simulink model "profinet_simulation_ss_separated"  (R2016b)
settings: Solver=FixedStepAuto  StartTime=0.0  StopTime=80  FixedStep=Ts  RelTol=1e-3
values from neighbouring files (symbols this model uses):
  A = [0 1 0 ... (first row only)    [motor.m]
  B = [0 ; 0 ; 1/L]    [motor.m]
  C = [1 0 0]    [motor.m]
  K = dlqr(Gd.a,Gd.b,diag([1,1,1]),1)    [motor.m]
  Ts = 1e-3    (= 0.001)    [TimeDelayEstimationSearch_Profibus.m]    (also in motor.m = 0.0001)
  Ts_IRT = 1e-4    (= 0.0001)    [motor.m]
  Ts_RT = 1e-3    (= 0.001)    [TimeDelayEstimationSearch_Profibus.m]    (also in motor.m)
  Ts_SRT = 1e-1    (= 0.1)    [motor.m]
libraries: simulink x4
settings Model: Creator=z003vh9b  LastModifiedBy=z003vh9b
settings OptimizationCC: BlockReduction=off  DefaultParameterBehavior=Inlined  BufferReuse=off

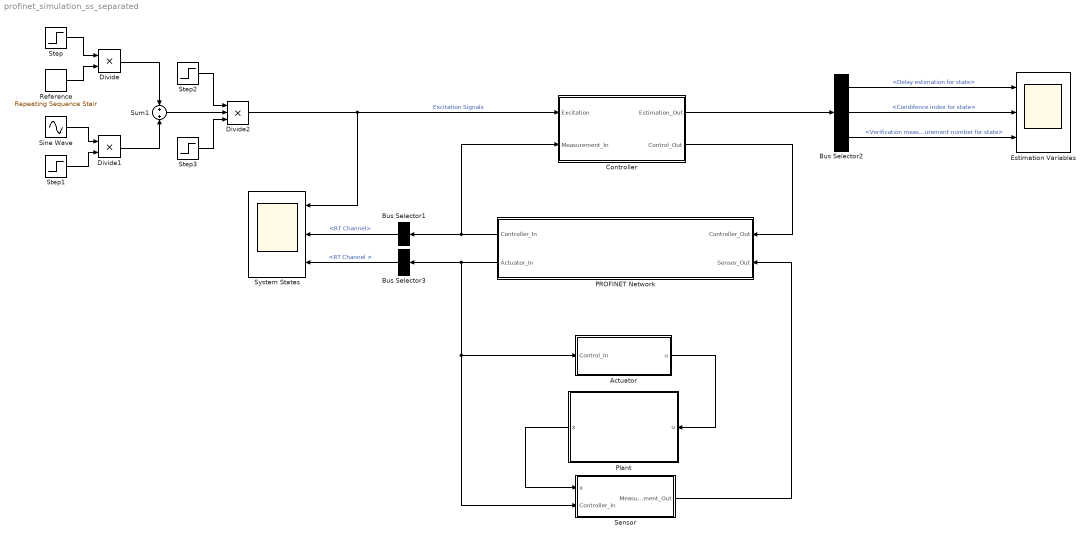
== system profinet_simulation_ss_separated ==
  Actuator : Subsystem  mask(Actuator with PROFIBUS interface){Gain=1, ActuatorCh=RT}
      mask prompts: Gain "Control Gain - Signal Conversion"; ActuatorCh "Control Signal Channel"
      mask help: Actuator Device connected to PROFIBUS network connection.
      mask TypeOptions ActuatorCh: RT | IRT
  Bus Selector1 : BusSelector  OutputSignals=RT Channel
  Bus Selector2 : BusSelector  OutputSignals=Delay estimation for state,Condifence index for state,Verification measurement number for state
  Bus Selector3 : BusSelector  OutputSignals=RT Channel
  Controller : Subsystem  mask(Controller Device with PROFINET Interface){K=K, SensorCh=RT, ActuatorCh=RT, N_ver=90}
      mask prompts: K "Gain"; SensorCh "Sensor measurement Channel"; ActuatorCh "Actuator control Channel"; N_ver "Verification Buffer Size (n samples)"
      mask help: Controller device connected to PROFINET network sending actuator control signals and receiving sensor measurements. Closed loop control is done as State-space optimal control.
      mask TypeOptions SensorCh: RT | IRT
      mask TypeOptions ActuatorCh: RT | IRT
  Divide : Product  Inputs=**
  Divide1 : Product  Inputs=**
  Divide2 : Product  Inputs=***
  Estimation Variables : Scope  NumInputPorts=3
  PROFINET Network : Subsystem  mask(PROFINET network simulation with attacks){PckgLossRate=20, PckgTimeLow=30, PckgTimeUp=90, AttackSensorRT=on, T_RT_Att_Sen=[7.8 2.1 5.04], Val_RT_Att_Sen_init=[0 0 0], Val_RT_Att_Sen=[6 12 10], AttackSensorIRT=off, T_IRT_Att_Sen=0, Val_IRT_Att_Sen_init=0, Val_IRT_Att_Sen=500, AttackControlRT=off, T_RT_Att_Cnt=5, Val_RT_Att_Cnt=3, AttackControlIRT=off, T_IRT_Att_Cnt=3, Val_IRT_Att_Cnt=-2}
      mask prompts: PckgLossRate "Package loss Rate [%]"; PckgTimeLow "Package arival time variation Lower litmit [%] 0-100% Ts"; PckgTimeUp "Package arival time variation Upper litmit [%] 0-100%Ts"; AttackSensorRT "RT Measurement Channel Attack"; T_RT_Att_Sen "Time of the Attack [s]"; Val_RT_Att_Sen_init "Initial Delay Value (n sampling times)"; Val_RT_Att_Sen "Delay Value (n sampling times)"; AttackSensorIRT "IRT Measurement Channel Attack"; T_IRT_Att_Sen "Time of the Attack [s]"; Val_IRT_Att_Sen_init "Initial Delay Value (n sampling times)"; Val_IRT_Att_Sen "Delay Value (n sampling times)"; AttackControlRT "RT Control Channel Attack"; T_RT_Att_Cnt "Time of the Attack [s]"; Val_RT_Att_Cnt "Attack Control Value [V]"; AttackControlIRT "IRT Control Channel Attack"; T_IRT_Att_Cnt "Time of the Attack [s]"; Val_IRT_Att_Cnt "Attack Control Value [V]"
      mask help: This block represents PROFINET network simulaiton with configulable packet loss and time delays. Additionally simulation of Man in the middle cyber attack is provided on both sensor measuremnt side as well as actuator control value.
  Plant : Subsystem  mask(Plant){A=A, B=B, C=C, x0=0}
      mask prompts: A "A Matrix"; B "B Matrix"; C "C Matrix"; x0 "Xo"
      mask help: This dynamical LTI system does not have awareness of PROFINET network. It is formed as continous State-Space domain and all the states can be measured and are provided at the output port (x).
  Reference : simulink/Sources/Repeating Sequence Stair  OutValues=[0 1 2 1 -1].'  tsamp=2  OutMin=[]  OutMax=[]  OutDataTypeStr=double  OutputDataTypeScalingMode=double  OutDataType=fixdt(0,8)  ConRadixGroup=Best Precision: Vector-wise  OutScaling=2^-12
  Sensor : Subsystem  mask(Sensor with PROFIBUS interface){SensorGain=[1 1 1], QuantizationEnable=on, SensorQuantMax=[1 1 1], SensorQuantMin=[-1 -1 -1], SensorQuantN=[2000 2000 2000], SensorNoise=on, NoiseMagnitude=[1e-3 1e-3 1e-3], SensorCh=RT, N_samples=30}
      mask prompts: SensorGain "Sensor Gain - Signal Conversion"; QuantizationEnable "Enable Quantization"; SensorQuantMax "Sensor State Max"; SensorQuantMin "Sensor State Min"; SensorQuantN "Sensor State Quantization - N"; SensorNoise "Enable Smart Noise"; NoiseMagnitude "Smart Noise Unit Magnitude"; SensorCh "Sensor Measurement Channel"; N_samples "Maximal Verification Measurement Number ( n samples )"
      mask help: Sensor Device connected to PROFIBUS network connection. It sends all state variables posible to meassure to the Controller Device.
      mask TypeOptions SensorCh: RT | IRT
      mask DialogControl Control2 Prompt: Sensor states quantiosation (Max-Min)/N
  Sine Wave : Sin  Amplitude=[1 1 1]  Frequency=[70*pi, 60*pi,80*pi]  SampleTime=0
  Step : Step  Time=20  Before=1  After=0  SampleTime=0
  Step1 : Step  Time=40  SampleTime=0
  Step2 : Step  Time=60  Before=1  After=0  SampleTime=0
  Step3 : Step  Time=0  SampleTime=0
  Sum1 : Sum
  System States : Scope  NumInputPorts=3
  wires:
  Actuator/1(u) -> Plant/1(u)
  PROFINET Network/1(Controller_In) -> Controller/2(Measurement_In), Bus Selector1/1
  Plant/1(x) -> Sensor/1(x)
  Controller/2(Control_Out) -> PROFINET Network/1(Controller_Out)
  Sensor/1(Measurement_Out) -> PROFINET Network/2(Sensor_Out)
  PROFINET Network/2(Actuator_In) -> Sensor/2(Controller_In), Actuator/1(Control_In), Bus Selector3/1
  Bus Selector1/1 -> System States/2  "<RT Channel>"
  Controller/1(Estimation_Out) -> Bus Selector2/1
  Bus Selector2/2 -> Estimation Variables/2  "<Condifence index for state>"
  Bus Selector2/1 -> Estimation Variables/1  "<Delay estimation for state>"
  Bus Selector2/3 -> Estimation Variables/3  "<Verification measurement number for state>"
  Bus Selector3/1 -> System States/3  "<RT Channel >"
  Sum1/1 -> Divide2/2
  Sine Wave/1 -> Divide1/1
  Reference/1 -> Divide/2
  Divide1/1 -> Sum1/2
  Divide/1 -> Sum1/1
  Divide2/1 -> Controller/1(Excitation), System States/1  "Excitation Signals"
  Step/1 -> Divide/1
  Step1/1 -> Divide1/2
  Step2/1 -> Divide2/1
  Step3/1 -> Divide2/3

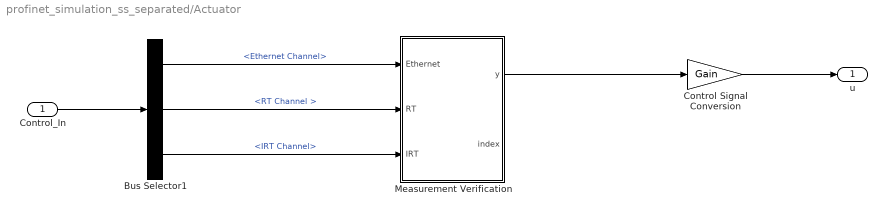
== system profinet_simulation_ss_separated/Actuator ==
  Control_In : Inport
  Bus Selector1 : BusSelector  OutputSignals=Ethernet Channel,RT Channel ,IRT Channel
  Control Signal Conversion : Gain  Gain=Gain
  Measurement Verification : MATLAB Function  TreatAsAtomicUnit=on
  u : Outport
  wires:
  Measurement Verification/1(y) -> Control Signal Conversion/1
  Bus Selector1/3 -> Measurement Verification/3(IRT)  "<IRT Channel>"
  Bus Selector1/1 -> Measurement Verification/1(Ethernet)  "<Ethernet Channel>"
  Control Signal Conversion/1 -> u/1
  Control_In/1 -> Bus Selector1/1
  Bus Selector1/2 -> Measurement Verification/2(RT)  "<RT Channel >"

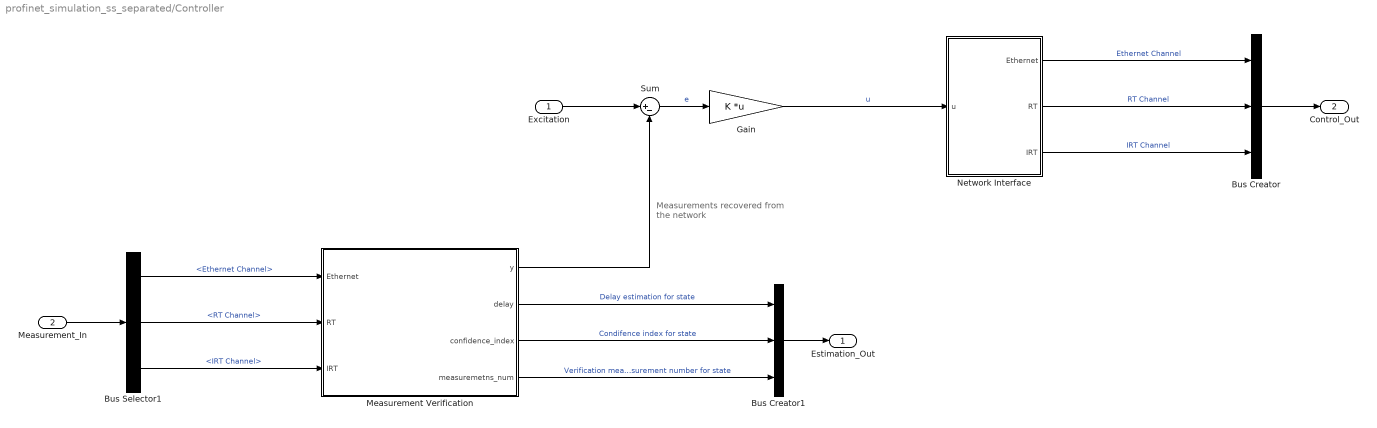
== system profinet_simulation_ss_separated/Controller ==
  note: Measurements recovered
      | from the network
  Excitation : Inport
  Measurement_In : Inport  Port=2
  Bus Creator : BusCreator  Inputs=3
  Bus Creator1 : BusCreator  Inputs=3
  Bus Selector1 : BusSelector  OutputSignals=Ethernet Channel,RT Channel,IRT Channel
  Gain : Gain  Gain=K  Multiplication=Matrix(K*u) (u vector)
  Measurement Verification : MATLAB Function  TreatAsAtomicUnit=on  SystemSampleTime=Ts
  Network Interface : MATLAB Function  TreatAsAtomicUnit=on  SystemSampleTime=Ts
  Sum : Sum  Inputs=|+-
  Estimation_Out : Outport
  Control_Out : Outport  Port=2
  wires:
  Sum/1 -> Gain/1  "e"
  Measurement Verification/1(y) -> Sum/2
  Gain/1 -> Network Interface/1(u)  "u"
  Network Interface/2(RT) -> Bus Creator/2  "RT Channel"
  Bus Selector1/1 -> Measurement Verification/1(Ethernet)  "<Ethernet Channel>"
  Bus Selector1/2 -> Measurement Verification/2(RT)  "<RT Channel>"
  Bus Selector1/3 -> Measurement Verification/3(IRT)  "<IRT Channel>"
  Network Interface/1(Ethernet) -> Bus Creator/1  "Ethernet Channel"
  Network Interface/3(IRT) -> Bus Creator/3  "IRT Channel"
  Measurement Verification/2(delay) -> Bus Creator1/1  "Delay estimation for state"
  Measurement Verification/3(confidence_index) -> Bus Creator1/2  "Condifence index for state"
  Measurement Verification/4(measuremetns_num) -> Bus Creator1/3  "Verification measurement number for state"
  Bus Creator/1 -> Control_Out/1
  Measurement_In/1 -> Bus Selector1/1
  Bus Creator1/1 -> Estimation_Out/1
  Excitation/1 -> Sum/1

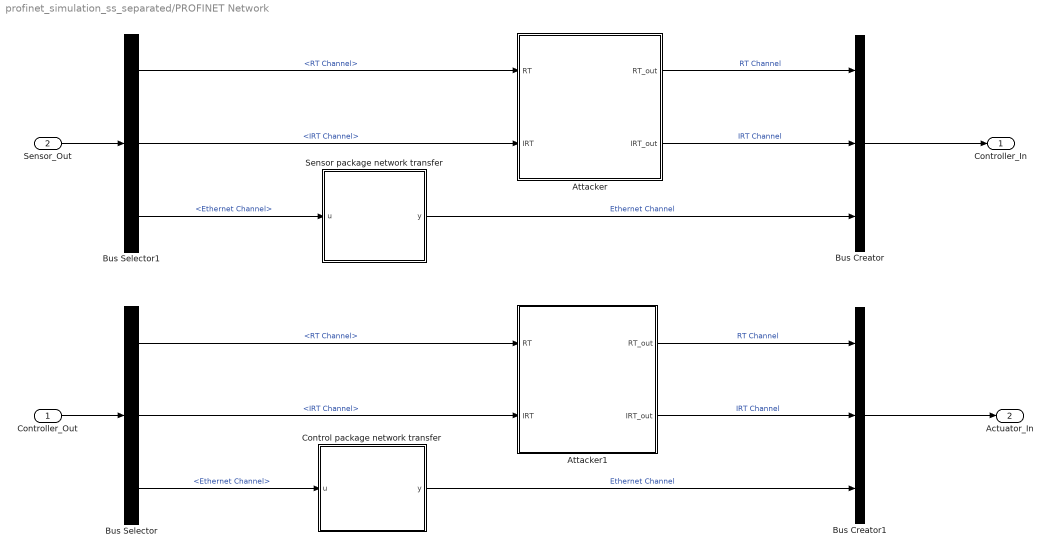
== system profinet_simulation_ss_separated/PROFINET Network ==
  Controller_Out : Inport
  Sensor_Out : Inport  Port=2
  Attacker : Subsystem
  Attacker1 : Subsystem
  Bus Creator : BusCreator  Inputs=3
  Bus Creator1 : BusCreator  Inputs=3
  Bus Selector : BusSelector  OutputSignals=RT Channel,IRT Channel,Ethernet Channel
  Bus Selector1 : BusSelector  OutputSignals=RT Channel,IRT Channel,Ethernet Channel
  Control package network transfer : MATLAB Function  TreatAsAtomicUnit=on
  Sensor package network transfer : MATLAB Function  TreatAsAtomicUnit=on
  Controller_In : Outport
  Actuator_In : Outport  Port=2
  wires:
  Attacker/1(RT_out) -> Bus Creator/1  "RT Channel"
  Attacker1/1(RT_out) -> Bus Creator1/1  "RT Channel"
  Bus Selector/1 -> Attacker1/1(RT)  "<RT Channel>"
  Control package network transfer/1(y) -> Bus Creator1/3  "Ethernet Channel"
  Sensor package network transfer/1(y) -> Bus Creator/3  "Ethernet Channel"
  Controller_Out/1 -> Bus Selector/1
  Bus Selector/3 -> Control package network transfer/1(u)  "<Ethernet Channel>"
  Sensor_Out/1 -> Bus Selector1/1
  Bus Creator/1 -> Controller_In/1
  Bus Creator1/1 -> Actuator_In/1
  Bus Selector1/2 -> Attacker/2(IRT)  "<IRT Channel>"
  Bus Selector1/3 -> Sensor package network transfer/1(u)  "<Ethernet Channel>"
  Bus Selector1/1 -> Attacker/1(RT)  "<RT Channel>"
  Attacker/2(IRT_out) -> Bus Creator/2  "IRT Channel"
  Bus Selector/2 -> Attacker1/2(IRT)  "<IRT Channel>"
  Attacker1/2(IRT_out) -> Bus Creator1/2  "IRT Channel"

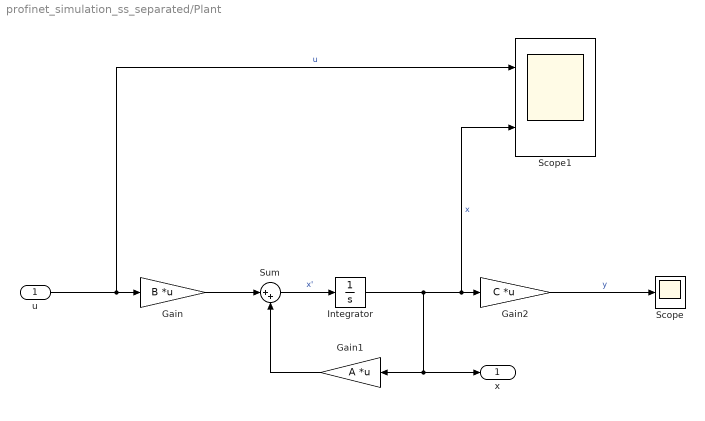
== system profinet_simulation_ss_separated/Plant ==
  u : Inport
  Gain : Gain  Gain=B  Multiplication=Matrix(K*u) (u vector)
  Gain1 : Gain  Gain=A  Multiplication=Matrix(K*u)
  Gain2 : Gain  Gain=C  Multiplication=Matrix(K*u) (u vector)
  Integrator : Integrator  InitialCondition=x0
  Scope : Scope
  Scope1 : Scope  NumInputPorts=2
  Sum : Sum  Inputs=|++
  x : Outport
  wires:
  u/1 -> Scope1/1, Gain/1  "u"
  Integrator/1 -> Gain1/1, x/1, Scope1/2, Gain2/1  "x"
  Gain1/1 -> Sum/2
  Sum/1 -> Integrator/1  "x'"
  Gain/1 -> Sum/1
  Gain2/1 -> Scope/1  "y"

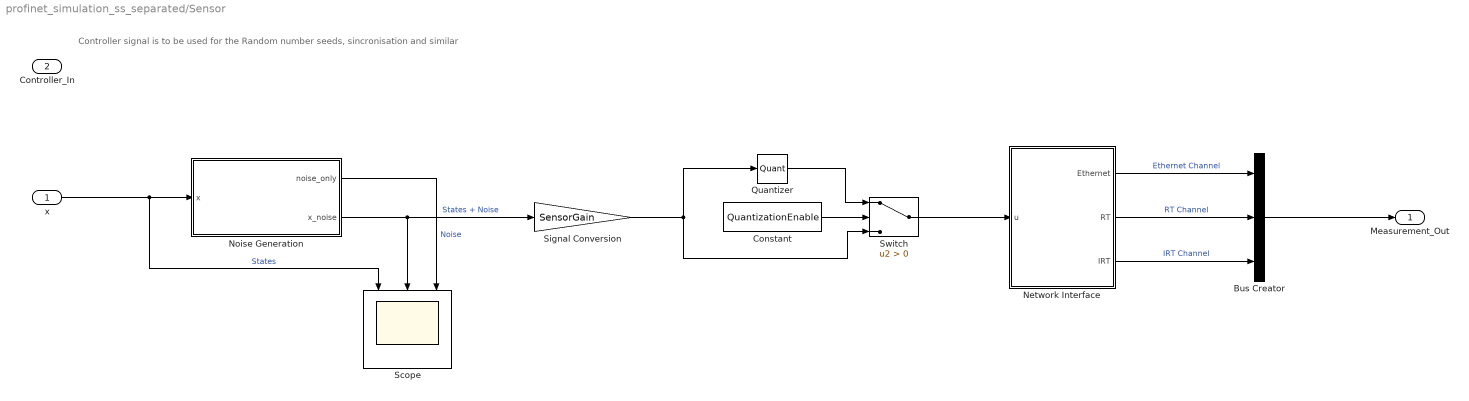
== system profinet_simulation_ss_separated/Sensor ==
  note: Controller signal is to be used for the Random number seeds, sincronisation and similar
  x : Inport
  Controller_In : Inport  Port=2
  Bus Creator : BusCreator  Inputs=3
  Constant : Constant  Value=QuantizationEnable
  Network Interface : MATLAB Function  TreatAsAtomicUnit=on  SystemSampleTime=Ts
  Noise Generation : MATLAB Function  TreatAsAtomicUnit=on  SystemSampleTime=Ts
  Quantizer : Quantizer  QuantizationInterval=(SensorQuantMax-SensorQuantMin)./SensorQuantN
  Scope : Scope  NumInputPorts=3
  Signal Conversion : Gain  Gain=SensorGain
  Switch : Switch  Criteria=u2 > Threshold
  Measurement_Out : Outport
  wires:
  Network Interface/2(RT) -> Bus Creator/2  "RT Channel"
  Network Interface/1(Ethernet) -> Bus Creator/1  "Ethernet Channel"
  Noise Generation/2(x_noise) -> Signal Conversion/1, Scope/2  "States + Noise"
  Network Interface/3(IRT) -> Bus Creator/3  "IRT Channel"
  x/1 -> Noise Generation/1(x), Scope/1  "States"
  Signal Conversion/1 -> Switch/3, Quantizer/1
  Switch/1 -> Network Interface/1(u)
  Quantizer/1 -> Switch/1
  Constant/1 -> Switch/2
  Bus Creator/1 -> Measurement_Out/1
  Noise Generation/1(noise_only) -> Scope/3  "Noise"

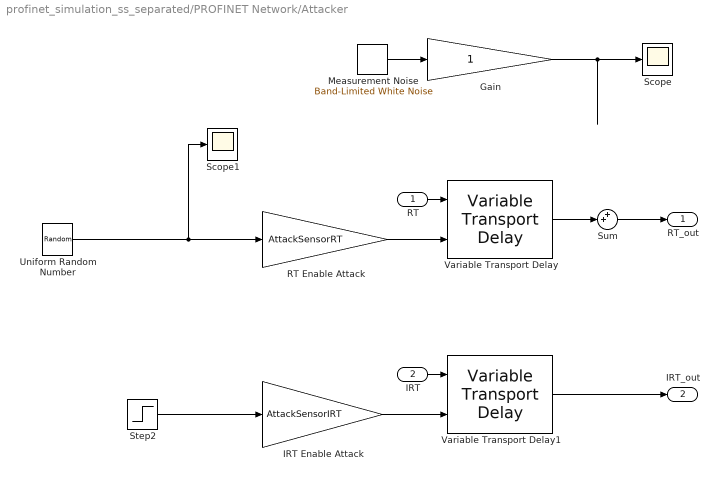
== system profinet_simulation_ss_separated/PROFINET Network/Attacker ==
  RT : Inport  PortDimensions=3
  IRT : Inport  Port=2  PortDimensions=3
  Gain : Gain
  IRT Enable Attack : Gain  Gain=AttackSensorIRT
  Measurement Noise : simulink/Sources/Band-Limited White Noise  Cov=[10e-3,10e-3,10e-3].^2* Ts/(2*pi)  Ts=Ts  seed=[432,23534653441,2353234]
  RT Enable Attack : Gain  Gain=AttackSensorRT
  Scope : Scope
  Scope1 : Scope
  Step2 : Step  Time=T_IRT_Att_Sen  Before=Val_IRT_Att_Sen_init*Ts_RT  After=Val_IRT_Att_Sen*Ts_RT  SampleTime=0
  Sum : Sum  Inputs=++|
  Uniform Random Number : UniformRandomNumber  Minimum=[0,0,0]  Maximum=Val_RT_Att_Sen*Ts_RT  Seed=[0,40,7]  SampleTime=7.7
  Variable Transport Delay : VariableTransportDelay  MaximumDelay=10  InitialOutput=[0 0 0]  ZeroDelay=on
  Variable Transport Delay1 : VariableTransportDelay  MaximumDelay=10  ZeroDelay=on
  RT_out : Outport
  IRT_out : Outport  Port=2
  wires:
  RT Enable Attack/1 -> Variable Transport Delay/2
  RT/1 -> Variable Transport Delay/1
  Variable Transport Delay/1 -> Sum/2
  Variable Transport Delay1/1 -> IRT_out/1
  IRT Enable Attack/1 -> Variable Transport Delay1/2
  IRT/1 -> Variable Transport Delay1/1
  Step2/1 -> IRT Enable Attack/1
  Measurement Noise/1 -> Gain/1
  Gain/1 -> Scope/1
  Sum/1 -> RT_out/1
  Uniform Random Number/1 -> Scope1/1, RT Enable Attack/1

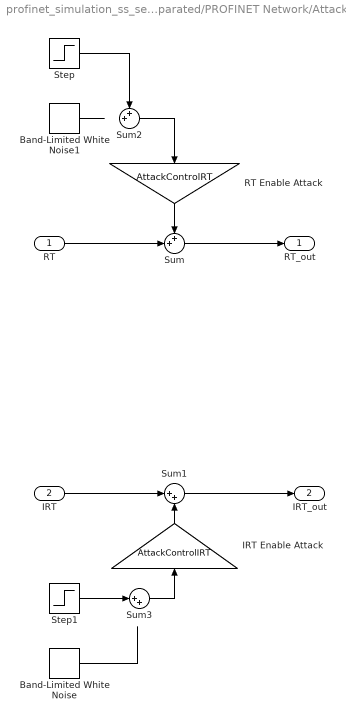
== system profinet_simulation_ss_separated/PROFINET Network/Attacker1 ==
  RT : Inport
  IRT : Inport  Port=2
  Band-Limited White Noise : simulink/Sources/Band-Limited White Noise  Cov=5e-7  Ts=0.001  seed=[241]
  Band-Limited White Noise1 : simulink/Sources/Band-Limited White Noise  Cov=[5e-6]  Ts=0.01  seed=[23341]
  IRT Enable Attack : Gain  Gain=AttackControlIRT
  RT Enable Attack : Gain  Gain=AttackControlRT
  Step : Step  Time=T_RT_Att_Cnt  After=Val_RT_Att_Cnt  SampleTime=0
  Step1 : Step  Time=T_IRT_Att_Cnt  After=Val_IRT_Att_Cnt  SampleTime=0
  Sum : Sum  Inputs=++|
  Sum1 : Sum  Inputs=|++
  Sum2 : Sum  Inputs=++|
  Sum3 : Sum  Inputs=|++
  RT_out : Outport
  IRT_out : Outport  Port=2
  wires:
  Band-Limited White Noise1/1 -> ?
  Sum1/1 -> IRT_out/1
  IRT/1 -> Sum1/1
  RT/1 -> Sum/2
  Sum/1 -> RT_out/1
  Step/1 -> Sum2/1
  Step1/1 -> Sum3/1
  Band-Limited White Noise/1 -> ?
  RT Enable Attack/1 -> Sum/1
  Sum2/1 -> RT Enable Attack/1
  IRT Enable Attack/1 -> Sum1/2
  Sum3/1 -> IRT Enable Attack/1

== matlab function profinet_simulation_ss_separated/Actuator/Measurement Verification ==
  data: Ethernet input; y output; RT input; IRT input; index output; ActuatorCh parameter
function [y,index]= fcn(Ethernet, RT, IRT, ActuatorCh)

EncCh = Ethernet;
persistent y_SRT;
%% Initialisation
if isempty(y_SRT)
    y_SRT= 0;
end

%%  Sensor data is accepted via the PROFIBUS channel RT or IRT 
if ActuatorCh == 1
    y = RT;
else
    y = IRT;
end


%% Signal verification of SRT package receival
% if length(EncCh) > 1 && EncCh(2)
%       y_SRT = EncCh(1);
% end
index = [y_SRT];

== matlab function profinet_simulation_ss_separated/Controller/Network Interface ==
  data: u input; Ethernet output; RT output; IRT output; Ts_IRT parameter; Ts_RT parameter; Ts parameter; Ts_SRT parameter; ActuatorCh parameter
function [Ethernet, RT, IRT] = fcn(u, Ts_IRT, Ts_RT, Ts, Ts_SRT, ActuatorCh)

persistent t RT_old SRT_old IRT_old;
%% Initialisation
if isempty(t) 
    t=0;
    RT_old=zeros(length(u),1);
    IRT_old=zeros(length(u),1);
    SRT_old=zeros(length(u),1);
else
    t=t+1;
end

%% Multiplexing data in three PROFINET channels 
%
%  The data control data is sent either by RT or IRT channel and SRT
%  channel is used to verify sent data to prevent cyber attacks
%
% IRT
if mod(t,floor(Ts_IRT/Ts)) == 0  && ActuatorCh == 2
    IRT = u;
else
    IRT = IRT_old;
end
IRT_old=IRT;

% RT
if mod(t,floor(Ts_RT/Ts)) == 0 && ActuatorCh == 1
    RT = u;
else
    RT = RT_old;
end
RT_old=RT;

% SRT
if mod(t,floor(Ts_SRT/Ts)) == 0 
    Ethernet = [u, ones(length(u),1)];
else
    Ethernet = [SRT_old, zeros(length(u),1)];
end
SRT_old=Ethernet(1:length(u),1);

== matlab function profinet_simulation_ss_separated/PROFINET Network/Control package network transfer ==
  data: u input; y output; PckgTimeLow parameter; PckgTimeUp parameter; PckgLossRate parameter; Ts parameter; Ts_SRT parameter
function y  = fcn(u, PckgTimeLow, PckgTimeUp, PckgLossRate, Ts, Ts_SRT)

u_ = u;


persistent delay loss PckgLow PckgUp;

if isempty(delay)
    delay = zeros(length(u),1) - 1;
    loss = zeros(length(u),1) - 1;
    rng(3453426245);
    PckgLow = PckgTimeLow/100*round(Ts_SRT / Ts);
    PckgUp = PckgTimeUp/100*round(Ts_SRT / Ts);
end



len=length(u(:,1));
for i = 1: len
    if u(i,2) == 1
        delay(i) = round(PckgLow + (PckgUp-PckgLow)*rand(1));
        loss(i) = 100*rand(1);
        if loss(i) <= PckgLossRate
            delay(i) = -1;
        end
        u_(i,2) = 0;
    end
    
    if delay(i) > 0 
        delay(i) = delay(i) -1;
    elseif delay(i) == 0 
        delay(i) = -1;
        u_(i,2) = 1;
    end
end
y = u_;

== matlab function profinet_simulation_ss_separated/Sensor/Noise Generation ==
  data: noise_only output; x_noise output; SensorNoise parameter; NoiseMagnitude parameter; Ts_IRT parameter; Ts_RT parameter; Ts parameter; Ts_SRT parameter; x input; SensorCh parameter
function [noise_only,   x_noise]= fcn(SensorNoise,NoiseMagnitude,Ts_IRT, Ts_RT, Ts, Ts_SRT, x, SensorCh)


if ~SensorNoise 
    x_noise = x;
    noise_only = zeros(length(x),1);
    return;
end


persistent t noise ms register uniqueLength stages weights;
%% Initialisation
if isempty(t) 
    t=0;
    noise = zeros(length(x),1);
       
    % Random number algorithm intitialization 
    stages = 5;
    uniqueLength = 5;
    weights=[0, 0, 0, 1, 2];

%     baseVal = 3;
%     powerVal = 5;
%     weights=[1,1,2,0,2];

%     baseVal = 3;
%     powerVal = 7;
%     weights=[0,2,2,1,2,2,2];
    
    register=round(stages*rand(length(x),uniqueLength));

else
    t=t+1;
    
    if ~mod(t,Ts_SRT/Ts)
        % Re-inti value of the shiftReg every step of the Ethernet package
        % sent
    end
    
    % smart stuff RT
    if ~mod(t,Ts_RT/Ts) && SensorCh == 1
        
        ms=rem(register*weights'+stages,stages);
        register=[ms, register(:,1:uniqueLength-1)];
        noise = NoiseMagnitude'.* (ms - floor(stages/2-1)); % eg. 5 stages 0 1 2 3 4 5 -> -2 -1 0 1 2
    elseif  ~mod(t,Ts_IRT/Ts) && SensorCh == 2
        % smart stuff IRT


    end
end

noise_only = noise;
x_noise = x + noise;
end

function b = bipolar(a)
b = 2*a-1;
end

== matlab function profinet_simulation_ss_separated/Controller/Measurement Verification ==
  data: Ethernet input; y output; RT input; IRT input; delay output; SensorCh parameter; Ts_RT parameter; Ts_SRT parameter; Ts_IRT parameter; Ts parameter; N_ver parameter; confidence_index output; measuremetns_num output
function [y,delay,confidence_index,measuremetns_num] = fcn(Ethernet, RT, IRT, SensorCh, Ts_RT, Ts_SRT, Ts_IRT, Ts, N_ver)


persistent RT_buf IRT_buf delay_ind conf_ind t RT_snap_buf IRT_snap_buf N_samples_used measur_num;
%% Initialization
if isempty(t)
    RT_snap_buf = zeros(length(RT),N_ver);
    IRT_snap_buf = zeros(length(IRT),N_ver);
    RT_buf = zeros(length(RT),N_ver);
    IRT_buf = zeros(length(IRT),N_ver);
    delay_ind = zeros(length(Ethernet(:,1)),1);
    conf_ind = zeros(length(Ethernet(:,1)),1);
    measur_num = zeros(length(Ethernet(:,1)),1);
    t = 0;
    N_samples_used = 5*ones(length(Ethernet(:,1)),3);
else
    t=t+1;
    if ~mod(t,floor(Ts_SRT/Ts))
        if SensorCh == 1
            RT_snap_buf = RT_buf;
        elseif  SensorCh == 2
            IRT_snap_buf = IRT_buf;
        end
    else
        if (mod(t,floor(Ts_SRT/Ts)) <= (N_ver+1)*Ts_RT/Ts+1 && SensorCh == 1) || (mod(t,floor(Ts_SRT/Ts)) <= (N_ver+1)*Ts_IRT/Ts+1 && SensorCh == 2)
            if ~mod(t,Ts_RT/Ts) && SensorCh == 1
                RT_buf = [RT, RT_buf(:,1:N_ver-1)];
            elseif  ~mod(t,Ts_IRT/Ts) && SensorCh == 2
                IRT_buf = [IRT, IRT_buf(:,1:N_ver-1)];
            end
        end
    end
end

%%  Sensor data is accepted via PROFIBUS channel RT or IRT 
if SensorCh == 1
    y = [RT;zeros(3-length(RT),1)];
else
    y = [IRT;zeros(3-length(IRT),1)];
end

%% Signal verification upon receiving Etherent package 
for i = 1:length(Ethernet(:,1))
    if Ethernet(i,1)
        if SensorCh == 1
            %[ind(i,:), num(i,:)] = findDelaySamplingBurstExact(RT_snap_buf(i,:), Ethernet(i,2:end),i);
            %[delay_ind(i,:), conf_ind(i,:)] = findDelaySamplingBurst(RT_snap_buf(i,:), Ethernet(i,2:7),i);
            [delay_ind(i,:), conf_ind(i,:), measur_num(i,:)] = findDelayElnagar(RT_snap_buf(i,:), Ethernet(i,2:end),i);
        else
            [delay_ind(i,:), conf_ind(i,:)] = findDelaySamplingBurstExact(IRT_snap_buf(i,:), Ethernet(i,2:N_samples_used(i)),i);
        end
    end
end

delay =  delay_ind;
confidence_index =  conf_ind;
measuremetns_num = measur_num;

end


function [ind, n] = findDelaySamplingBurstExact(y_rt,y_eth,state)
    % Helping variables initialization
    s_max =  0;
    index = -1;
    
    persistent index_old max_index;
    if isempty(index_old)
        index_old = [-1 -1 -1];
        % Maximal time delay value/index that can be estimated
        % basically N_ver - N_samples + 1 
        max_index = length(y_rt)-length(y_eth)+1;
    end
    
    % The algorithm performs iterative search shifting y_eth array and
    % comparing to y_rt array in with the length(y_eth) window size 
    %
    % The algorithm searches for exact same pattern of values/measurements 
    %
    % The number of same patterns in tracked to calcualte confidence index
    %
    % Additionally last index is saved and introduced as heuristic value to
    % the algorithm
    %
    n = 0;
    for i = 1:max_index
      s_tmp = y_rt(i:length(y_eth)-1+i)-y_eth(1:length(y_eth));
      s=sum(s_tmp==0);
      if abs(s) >= abs(s_max)
        % Keeping track of number of repetitions of y_eth measurements
        % pattern the controller buffer - to be used for estimation 
        % confidence index
        if s == length(y_eth)
            n = n + 1;
        end
        % heuristic part
        if  index_old(state) == i
            % 1.01 is empiric value
            s_max = s*1.01;
        else
            s_max = s;
        end
        index = i;
      end
    end
    ind = max_index - index;
    % if it's not the perfect matching return -1
    if abs(s_max) < length(y_eth)
        ind = -1;
    end
    index_old(state)=index;
end

function [ind,n] = findDelaySamplingBurst(y_rt,y_eth,state)
    % Helping variables initialization
    s_min =  inf;
    index = -1;
    
    persistent index_old max_index;
    if isempty(index_old)
        index_old = [-1 -1 -1];
        % Maximal time delay value/index that can be estimated
        % basically N_ver - N_samples + 1 
        max_index = length(y_rt)-length(y_eth)+1;
    end
    
    % The algorithm performs iterative search shifting y_eth array and
    % comparing to y_rt array in with the length(y_eth) window size
    %
    %
    % The minimal distance index is saved and it is the taken as time-dealy
    % estimate
    %
    % The number of same patterns in tracked to calcualte confidence index
    %
    % Additionally last index is saved and introduced as heuristic value to
    % the algorithm
    %
    n = 0;
    for i =  1 : max_index
      % Simple absolute distance calculation in between two arrays
      s=sum(abs(...
                y_rt( i:length(y_eth)-1+i ) - y_eth...
                ));
      
      if abs(s) <= abs(s_min)
        s_min = s;
        index = i;
        % heuristic part
        if  index_old(state) == i
            % 1e-2 is empiric value
            s_min = s_min - 1e-2;
        end
        % Keeping track of number of repetitions of y_eth measurements
        % pattern the controller buffer - to be used for estimation 
        % confidence index
        if s <= 0
            n = n + 1;
        end
      end
    end
    index_old(state)=index;
    ind = max_index - index;
end

function [ind, n, mn] = findDelayElnagar(ver_buffer,ver_window,state)
    % Helping variables initialisation
    Emin =  inf;
    index = -1;
    
    persistent J lambda max_index N_samples_used N_samples_time;
    if isempty(J)
        % Maximal time delay value/index that can be estimated
        % basically N_ver - N_samples + 1 
        max_index = length(ver_buffer)-length(ver_window)+1;
        
        % An performance index - algorithm searches for it's minimum
        J = zeros(max_index,3);
        % forgetting factor - Recursive estimation
        lambda = 0.01;
        
        N_samples_used = 10*ones(1,3);
        N_samples_time = zeros(1,3);
    end
    
    y_eth = ver_window(end - N_samples_used(state)+1:end);
    y_rt = ver_buffer(end - (max_index - 1 + N_samples_used(state) - 1) : end);
    
    %% This algorithm is as well very simple and for explanantion see: 
    % System Identification and Adaptive control Based on a Variable Regression for System Having Unknown Delay
    % A. Elnagar
    % Equation (11,12,13,14,15)
    % 
    % New Method for Delay Estimation
    % A. Elnagar
    %
    % The algorithm is based on iterative search to minimize performance
    % index criterion
    % 
    %
    % The number of same patterns in tracked to calcualte confidence index
    %
    %
    % In it's core, the algorithm is RLS and is used to estimate system
    % parameters, but in this case, we know exact output of the system and
    % therefore there is no need to estimate parameters and output
    % accordingly
    %
    n = 0;
    for ki = 1 : max_index
        % To improve the performance of this algrithm burst sampling in
        % introduced
        %
        % Algorithm minimizes criterium by calculating distance in between
        % array as in Burst sampling algorithm 
        % It becomes a lot more stable
         
        % Burst sampling   
        dY = (y_rt(ki:ki+length(y_eth)-1) - y_eth);
        J(ki,state) = lambda*J(ki,state) + sum(dY.^2);
        %J(ki,state) = lambda*J(ki,state) + sum((u(ki:ki+length(y_eth)-1).*dY).^2);
        
        % Just one value
        %J(ki) = lambda*J(ki) + sum(((y_rt(ki) - y_eth(1))).^2);
        %J(ki) = lambda*J(ki) + sum((u(ki).*(y_rt(ki) - y_eth(1))).^2);
        
        if J(ki,state) <= Emin
           Emin = J(ki,state);
           index = ki;
        end
        % Keeping track of number of repetitions of y_eth measurements
        % pattern the controller buffer - to be used for estimation 
        % confidence index
        if abs(dY) == 0
           n = n+1;
        end
    end
    ind = max_index - index;
    
    % Confidence index calcualtion
    
    % Measurement number calcualtion
      
    if(n == 1)
        N_samples_time(state) = N_samples_time(state) + 1;
        if ( N_samples_time(state) > 10)
            N_samples_used(state) = N_samples_used(state) - 1;
            N_samples_time(state) = 0;
        end
    else
        N_samples_used(state) = N_samples_used(state) + 1;
        N_samples_time(state) = 0;
    end
    
    if(N_samples_used(state) >=  length(ver_window))
         N_samples_used(state) = length(ver_window)-1;
    elseif(N_samples_used(state) <  3)
         N_samples_used(state) = 3;
    end
    mn = N_samples_used(state);
end

function [ind, n, mn] = findDelaySinopoli(ver_buffer,ver_window,state)
    % Fucntion testing Chi square test on the measurement verification
    % Window and buffe to deternim whether it has been changed. 
    %
    % Additionaly it searches for zerro value of the test to find the exact
    % vaue of time-delay - i the delat is time delay attack
    InjectedNoiseVariance = 10e-3;
    n  = 0;
    ind =0;
    % Chi squared test
    mn = sum((ver_buffer(1:length(ver_window))-ver_window).*InjectedNoiseVariance^-1.*(ver_buffer(1:length(ver_window))-ver_window));
    % Time delay index search
    for i = 1:length(ver_buffer)-length(ver_window)
        % Track the number of repetitions inside buffer
        if( sum((ver_buffer(i:length(ver_window)+i -1)-ver_window).*InjectedNoiseVariance^-1.*(ver_buffer(i:length(ver_window)+i -1)-ver_window)) == 0 )
           n = n+1;
           ind = i;
        end
    end
    % Value adaptation
    ind = length(ver_buffer)-length(ver_window) -ind;
end

== matlab function profinet_simulation_ss_separated/Sensor/Network Interface ==
  data: u input; Ethernet output; RT output; IRT output; Ts_IRT parameter; Ts_RT parameter; Ts parameter; Ts_SRT parameter; SensorCh parameter; N_samples parameter
function [Ethernet, RT, IRT] = fcn(u, Ts_IRT, Ts_RT, Ts, Ts_SRT, SensorCh, N_samples)

persistent t RT_old SRT_old IRT_old u_buf;
%% Initialisation
if isempty(t) 
    t=0;
    RT_old=zeros(length(u),1);
    IRT_old=zeros(length(u),1);
    SRT_old=zeros(length(u),N_samples);
    u_buf = zeros(length(u),N_samples);
    t=t+1;
else
    t=t+1;
    if mod(t,floor(Ts_SRT/Ts)) ~= 0
        if (mod(t,floor(Ts_SRT/Ts)) <= (N_samples+1)*Ts_RT/Ts+1 && SensorCh == 1) || (mod(t,floor(Ts_SRT/Ts)) <= (N_samples+1)*Ts_IRT/Ts+1 && SensorCh == 2)
            if ~mod(t,Ts_RT/Ts) && SensorCh == 1
                u_buf = [u, u_buf(:,1:N_samples-1)];
            elseif  ~mod(t,Ts_IRT/Ts) && SensorCh == 2
                u_buf = [u, u_buf(:,1:N_samples-1)];
            end
        end
    end
end

%% Multiplexing data in three PROFINET channels 
%
%  The data sensor data is sent either by RT or IRT channel and SRT
%  channel is used to verify sent data to prevent cyber attacks
%
% IRT
if mod(t,floor(Ts_IRT/Ts)) == 0  && SensorCh == 2
    IRT = u;
else
    IRT = IRT_old;
end
IRT_old=IRT;

% RT
if mod(t,floor(Ts_RT/Ts)) == 0 && SensorCh == 1
    RT = u;
else
    RT = RT_old;
end
RT_old=RT;

% SRT
if mod(t,floor(Ts_SRT/Ts)) == 0 
    Ethernet = [ones(length(u(:,1)),1),u_buf];
else
    Ethernet = [zeros(length(u(:,1)),1),SRT_old];
end
SRT_old=Ethernet(:,2:N_samples+1);

== matlab function profinet_simulation_ss_separated/PROFINET Network/Sensor package network transfer ==
  data: u input; y output; Ts_SRT parameter; PckgTimeLow parameter; PckgTimeUp parameter; PckgLossRate parameter; Ts parameter
function y  = fcn(u, Ts_SRT, PckgTimeLow, PckgTimeUp, PckgLossRate, Ts)

u_ = u;

persistent delay loss PckgLow PckgUp;

if isempty(delay)
    delay = zeros(length(u),1) - 1;
    loss = zeros(length(u),1) - 1;
    rng(345342645);
    PckgLow = PckgTimeLow/100*round(Ts_SRT / Ts);
    PckgUp = PckgTimeUp/100*round(Ts_SRT / Ts);
end



len=length(u(:,1));
for i = 1: len
    if u(i,1) == 1
        delay(i) = round(PckgLow + (PckgUp-PckgLow)*rand(1));
        loss(i) = 100*rand(1);
        if loss(i) <= PckgLossRate
            delay(i) = -1;
        end
        u_(i,1) = 0;
    end
    
    if delay(i) > 0 
        delay(i) = delay(i) -1;
    elseif delay(i) == 0 
        delay(i) = -1;
        u_(i,1) = 1;
    end
end
y = u_;
